simulink model "model_reentry"  (R2017b)
settings: Solver=VariableStepAuto  StartTime=0.0  StopTime=300  RelTol=1e-3
values from neighbouring files (symbols this model uses):
  xi = [v_ini, gamma_ini, h_ini, phi_ini, theta_ini, q_ini]    [load_to_simulink.m]    (also in reentry_simulator.m)
undefined symbols (not defined in the file or in its folder): Atm, Mars, sim_params, Vehicle
settings Model: Creator=Administrateur  LastModifiedBy=Administrateur

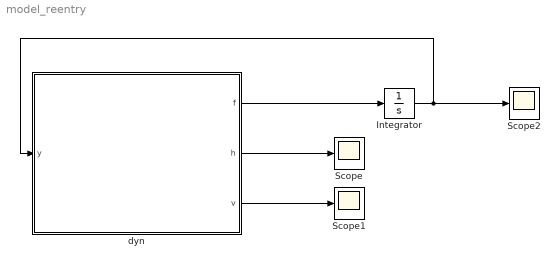
== system model_reentry ==
  Integrator : Integrator  InitialCondition=xi
  Scope : Scope
  Scope1 : Scope
  Scope2 : Scope
  dyn : MATLAB Function  TreatAsAtomicUnit=on
  wires:
  dyn/1(f) -> Integrator/1
  Integrator/1 -> dyn/1(y), Scope2/1
  dyn/2(h) -> Scope/1
  dyn/3(v) -> Scope1/1

== matlab function model_reentry/dyn ==
  data: f output; y input; Mars parameter; Atm parameter; Vehicle parameter; sim_params parameter; h output; v output
function [f, h, v] = Dynamics(y, Mars, Atm, Vehicle, sim_params)
    v = y(1);
    gamma = y(2);
    h = y(3);
    phi = y(4);
    theta = y(5);
    q = y(6);
    % m = y(5) To be implemented
    f = [0; 0; 0; 0; 0; 0];
    % Intermediate calculation
    r = h + Mars.radius * 1000;
    g = Mars.mu / r^2; % m/s^2 - Gravitationnal acceleration at r
    if h > 120000
        rho = 0;
    else
        rho =  Atm.rho0 * exp(-h/Atm.hs);
    end
    Pdyn = (1/2) * rho * (v^2 + 0.241^2); % Dynamic pressure

    
    if h < 10000
        t = -1.019e-11 * h.^3 + 1.349e-08 * h.^2 +...
            -1.958e-05 * h.^1 + 214; % K - Temperature
    elseif h >= 10000 && h <= 70000
        t = 2.845e-18 * h.^4 + -4.139e-13 * h.^3 + ...
              3.048e-08 * h.^2 -0.002304 * h.^1 + ...
              225.2; % K - Temperature
    elseif h > 70000 && h <= 100000
        t = 139; % K - Temperature
    else
        t = 0.001035 * h + 35.52; % K - Temperature
    end
    speed = sqrt(Atm.gamma * Atm.R * t);
    M = v ./ speed;
    alpha = theta - gamma;
    
    CA = CASimulink(M, alpha);
    CN = CNSimulink(M, alpha);
    
    CD = CA;
    CL = CD / (-20.833 * rad2deg(alpha));
    
    if (sim_params.controlled)
        B = CD * Vehicle.S / Vehicle.mass;
        dv_aero = sim_params.v_des - sqrt(v^2+((2*Mars.mu)*((1/sim_params.r_des)-(1/r))));
        gamma_ref = (1/2)*B*Atm.hs*((sim_params.rho_des - rho) ./ log(1 + dv_aero/v));
        
        k = (Pdyn * Vehicle.S * CL) / (v * Vehicle.mass); % equivalent to g
        theta_eq = gamma - (cos(gamma) * Vehicle.mass) / (Pdyn*Vehicle.S*CL) * (v^2/r - Mars.mu / r^2);
        theta_cmd = theta_eq + (1/(sim_params.tau*k)) * (gamma_ref - gamma);
        
        % saturation
        if (theta_cmd > deg2rad(60))
            theta_cmd = deg2rad(60);
        end
        
        Kp = sim_params.wn^2;
        Kd = 2 * sim_params.zeta * sim_params.wn;
        k = (Vehicle.CMdelta * Pdyn * Vehicle.S * Vehicle.d) / Vehicle.J;
        delta_eq = (-Vehicle.CMalpha/Vehicle.CMdelta) * (theta - gamma) - (Vehicle.CMq * Vehicle.d * q) / (2 * v * Vehicle.CMdelta);
        delta_cmd = delta_eq + Kp/k * (theta_cmd - theta) + Kd/k * (-q);
    else
        delta_cmd = 0;
    end
    
    
    Daero = Pdyn * Vehicle.S * CD;
    Laero = Daero / (-20.833 * rad2deg(alpha));
    Maero = Pdyn * Vehicle.S * Vehicle.d * (Vehicle.CMalpha * alpha + (Vehicle.d / (2*v)) * Vehicle.CMq*q + Vehicle.CMdelta * delta_cmd);
    
    if (h <= sim_params.parachute_at)
        Daero = Daero + Vehicle.Parachute.CD .* ((rho .* v.^2) / 2) * Vehicle.Parachute.S;
    end
    
    if (h <= 0)
        f(1) = 0;
    else
        f(1) = (-Daero) / Vehicle.mass - g*sin(gamma);
    end
    
    f(2) = (1/v) * (Laero/Vehicle.mass + ((v.^2/r) - g)*cos(gamma));
    
    if (h <= 0)
        f(3) = 0;
    else
        f(3) = v * sin(gamma);
    end
    f(4) = v/r * cos(gamma);
    f(5) = q;
    f(6) = (1 / Vehicle.J) * Maero;
    
    f = f(:);
end
